simulink model "moteur_cc_ass_vit_control_sys_des_tf"  (R2020a)
settings: Solver=ode15s  StartTime=0.0  StopTime=10  FixedStep=0.1  RelTol=1e-3  EnableMultiTasking=on
values from neighbouring files (symbols this model uses):
  f = 0.01    [parametres_moteur_cc.m]
  J = 0.015    [parametres_moteur_cc.m]
  Ke = 0.9    [parametres_moteur_cc.m]
  Km = 0.9    [parametres_moteur_cc.m]
  L = 0.4    [parametres_moteur_cc.m]
  R = 2    [parametres_moteur_cc.m]
settings Model: Creator=Ivan  LastModifiedBy=ivanl
settings DataIOCC: LimitDataPoints=on  SaveFormat=Array  SignalLoggingSaveFormat=ModelDataLogs  ReturnWorkspaceOutputs=off
settings OptimizationCC: ExpressionDepthLimit=2147483647  InitFltsAndDblsToZero=on  LifeSpan=inf
settings DebuggingCC: SaveWithParameterizedLinksMsg=none  UnderspecifiedInitializationDetection=Classic  MergeDetectMultiDrivingBlocksExec=none  SignalResolutionControl=TryResolveAllWithWarning  SolverPrmCheckMsg=warning  MultiTaskDSMMsg=warning  MultiTaskCondExecSysMsg=none  FcnCallInpInsideContextMsg=warning  AllowSymbolicDim=off  StateNameClashWarn=warning  SFUnexpectedBacktrackingDiag=warning  SFNoUnconditionalDefaultTransitionDiag=warning  SFExecutionAtInitializationDiag=none  ArithmeticOperatorsInVariantConditions=warning
settings HardwareCC: ProdBitPerPointer=32  ProdBitPerSizeT=32  ProdBitPerPtrDiffT=32  ProdLargestAtomicFloat=None  ProdIntDivRoundTo=Undefined  ProdEndianess=Unspecified  ProdWordSize=32  ProdHWDeviceType=32-bit Generic
settings ModelReferenceCC: PropagateSignalLabelsOutOfModel=off
settings SFSimCC: SimUseLocalCustomCode=off  CustomCodeUndefinedFunction=UseInterfaceOnly
settings RTWCC: RTWUseLocalCustomCode=off
settings CodeAppCC: StateflowObjectComments=on
settings GRTTargetCC: TargetFcnLib=ansi_tfl_tmw.mat  TargetLangStandard=C89/C90 (ANSI)  CombineOutputUpdateFcns=off  GRTInterface=on
settings ConfigComp: CovMetricSettings=dw  CovHtmlReporting=on  CovSaveCumulativeToWorkspaceVar=on  CovSaveSingleToWorkspaceVar=on  CovExternalEMLEnable=off

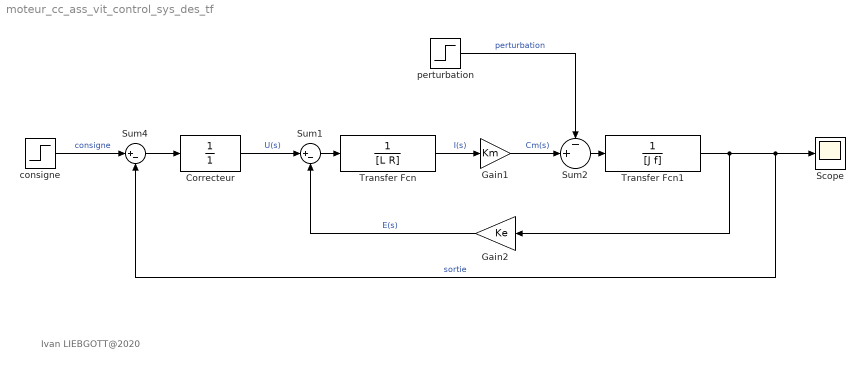
== system moteur_cc_ass_vit_control_sys_des_tf ==
  note: Ivan LIEBGOTT@2020
  Correcteur : TransferFcn  Denominator=[1]
  Gain1 : Gain  Gain=Km
  Gain2 : Gain  Gain=Ke
  Scope : Scope
  Sum1 : Sum  Inputs=|+-
  Sum2 : Sum  Inputs=-+|
  Sum4 : Sum  Inputs=|+-
  Transfer Fcn : TransferFcn  Denominator=[L R]
  Transfer Fcn1 : TransferFcn  Denominator=[J f]
  consigne : Step  Time=0  After=100  SampleTime=0
  perturbation : Step  Time=3  After=5  SampleTime=0
  wires:
  Sum1/1 -> Transfer Fcn/1
  Gain2/1 -> Sum1/2  "E(s)"
  Transfer Fcn/1 -> Gain1/1  "I(s)"
  Sum2/1 -> Transfer Fcn1/1
  perturbation/1 -> Sum2/1  "perturbation"
  Transfer Fcn1/1 -> Scope/1, Sum4/2, Gain2/1  "sortie"
  Sum4/1 -> Correcteur/1
  consigne/1 -> Sum4/1  "consigne"
  Gain1/1 -> Sum2/2  "Cm(s)"
  Correcteur/1 -> Sum1/1  "U(s)"
